simulink model "model"  (R2024b)
settings: Solver=ode1  StartTime=0.0  StopTime=10  FixedStep=0.0001  RelTol=1e-3
values from neighbouring files (symbols this model uses):
  a1 = c*a2    (= 810)    [init.m]
  a2 = c*a3    (= 270)    [init.m]
  a3 = c*a4    (= 90)    [init.m]
  a4 = c*10    (= 30)    [init.m]
  c1 = 50    [init.m]
  c2 = 1    [init.m]
  d = 100    [init.m]
  dis_gain = 30    [init.m]
  epsilon = 1    [init.m]
  i = 20    [init.m]
  k = 5    [init.m]
  mu = 0.9    [init.m]
  p = 400    [init.m]
  phi_frist = 0    [init.m]
  psi_frist = 0    [init.m]
  tau_p_max = 3000000    [init.m]
  theta_frist = 0    [init.m]
  umax = pi/2 - 0.01    (= 1.56079632679)    [init.m]
  w = wo    (= 50)    [init.m]
  wo = 50    [init.m]
  x_frist = 0    [init.m]
  y_frist = 0    [init.m]
  z_frist = 0    [init.m]
libraries: fod x36, slpidlib x6, simulink x1
(part 4 of 4)

== matlab function model/SMC/Subsystem/Subsystem6/MATLAB Function ==
  data: x input; z1_1 output; z1 input; z2 input; z3 input; z2_1 output; z3_1 output; z4 input; z4_1 output; a1 input; a2 input; a3 input; a4 input
function [z1_1,z2_1,z3_1,z4_1] = fcn(x,z1,z2,z3,z4,a1,a2,a3,a4)
    v1 = -a1*abs(z1-x)^(3/4)*sign(z1-x)+z2;
    z1_1 = v1;
    v2 = -a2*abs(z2-v1)^(2/3)*sign(z2-v1)+z3;
    z2_1 = v2;
    v3 = -a3*abs(z3-v2)^(1/2)*sign(z3-v2)+z4;
    z3_1 = v3;
    z4_1 = -a4*sign(z4-v3);
end

== matlab function model/MATLAB Function ==
  data: u input; y output
function y = fcn(u)

if u < 5
    y = 0;
else
    y = 1;
end

== matlab function model/系统5/MATLAB Function ==
  data: dnu output size=6*1; nu input; eta input; tau_p input; tau_d input; del input
function dnu = fcn(nu,eta,tau_p,tau_d,del)
    m = 5.5;
    I_x = 0.12;
    I_y = 0.25;
    I_z = 0.2;
    V = m;
    g = 9.8;

    x_B = 0;
    y_B = 0;
    z_B = -0.01;

    X_du = -2.61;
    K_dp = -0.15;
    X_u = -2.47;
    K_P = -0.82;
    X_uu = -8.33;
    K_pp = -2.95;
    Y_dv = -5.56;
    M_dq = -0.26;
    Y_v = -3.54;
    M_q = -0.9;
    Y_vv = -10.82;
    M_qq = -3.687;
    Z_dw = -9.75;
    N_dr = -0.21;
    Z_w = -2.38;
    N_r = -0.45;
    Z_ww = -14.13;
    N_rr = -1.56;

    m_u = m - X_du;
    m_v = m - Y_dv;
    m_w = m - Z_dw;
    m_p = I_x - K_dp;
    m_q = I_y - M_dq;
    m_r = I_z - N_dr;

    u = nu(1);
    v = nu(2);
    w = nu(3);
    p = nu(4);
    q = nu(5);
    r = nu(6);

    x = eta(1);
    y = eta(2);
    z = eta(3);
    phi = eta(4);
    theta = eta(5);
    psi = eta(6);

    M = [m_u 0 0 0 0 0;
         0 m_v 0 0 0 0;
         0 0 m_w 0 0 0;
         0 0 0 m_p 0 0;
         0 0 0 0 m_q 0;
         0 0 0 0 0 m_r];

    M = M+del*M;

    C = [0 0 0 0 m_w*w -m_r*v;
         0 0 0 -m_w*w 0 m_u*u;
         0 0 0 m_v*v -m_u*u 0;
         0 m_w*w -m_v*v 0 m_r*r -m_q*q;
         -m_w*w 0 m_u*u -m_r*r 0 m_p*p;
         m_v*v -m_u*u 0 m_q*q -m_p*p 0];

    C = C+del*C;
    
    D = -[X_uu*abs(u) 0 0 0 0 0;
          0 Y_vv*abs(v) 0 0 0 0;
          0 0 Z_ww*abs(w) 0 0 0;
          0 0 0 K_pp*abs(p) 0 0;
          0 0 0 0 M_qq*abs(q) 0;
          0 0 0 0 0 N_rr*abs(r)];

    D = D+del*D;
    
    B = g*V;

    g_eta = [0;0;0;-z_B*B*cos(theta)*sin(phi);-z_B*B*sin(theta);0];

    g_eta = g_eta+del*g_eta;

dnu = M\(tau_p + tau_d - C*nu - D*nu - g_eta);

== matlab function model/系统5/MATLAB Function1 ==
  data: eta input; deta output size=6*1; nv input
function deta = fcn(eta,nv)
    phi = eta(4);
    theta = eta(5);
    psi = eta(6);

    J =  [cos(psi)*cos(theta) -sin(psi)*cos(phi)+sin(phi)*sin(theta)*cos(psi) sin(psi)*sin(phi)+sin(theta)*cos(psi)*cos(phi) 0 0 0;
         sin(psi)*cos(theta) cos(psi)*cos(phi)+sin(phi)*sin(theta)*sin(psi) -cos(psi)*sin(phi)+sin(theta)*sin(psi)*cos(phi) 0 0 0;
         -sin(theta) sin(phi)*cos(theta) cos(psi)*cos(theta) 0 0 0;
         0 0 0 1 sin(phi)*tan(theta) cos(phi)*tan(theta);
         0 0 0 0 cos(phi) -sin(phi);
         0 0 0 0 sin(phi)/cos(theta) cos(phi)/cos(theta)];

deta = J*nv;

== matlab function model/ADRC/控制器/Subsystem1/Subsystem6/MATLAB Function2 ==
  data: h input; dh output size=3; eta input; tau_0 input; wo input
function dh = fcn(h,eta,tau_0,wo)

e = eta-h(1);

b1 = 3*wo;
b2  = 3*wo^2;
b3 = wo^3;

dh = [h(2)+b1*e;
    h(3)+b2*e+tau_0;
    b3*e;
    ];

== matlab function model/ADRC/控制器/Subsystem1/Subsystem1/MATLAB Function2 ==
  data: h input; dh output size=3; eta input; tau_0 input; wo input
function dh = fcn(h,eta,tau_0,wo)

e = eta-h(1);

b1 = 3*wo;
b2  = 3*wo^2;
b3 = wo^3;

dh = [h(2)+b1*e;
    h(3)+b2*e+tau_0;
    b3*e;
    ];

== matlab function model/FO_SMC_ESO/Levant微分器/Subsystem6/MATLAB Function ==
  data: x input; z1_1 output; z1 input; z2 input; z3 input; z2_1 output; z3_1 output; z4 input; z4_1 output; a1 input; a2 input; a3 input; a4 input
function [z1_1,z2_1,z3_1,z4_1] = fcn(x,z1,z2,z3,z4,a1,a2,a3,a4)
    v1 = -a1*abs(z1-x)^(3/4)*sign(z1-x)+z2;
    z1_1 = v1;
    v2 = -a2*abs(z2-v1)^(2/3)*sign(z2-v1)+z3;
    z2_1 = v2;
    v3 = -a3*abs(z3-v2)^(1/2)*sign(z3-v2)+z4;
    z3_1 = v3;
    z4_1 = -a4*sign(z4-v3);
end

== matlab function model/ADRC/控制器/Subsystem1/Subsystem2/MATLAB Function2 ==
  data: h input; dh output size=3; eta input; tau_0 input; wo input
function dh = fcn(h,eta,tau_0,wo)

e = eta-h(1);

b1 = 3*wo;
b2  = 3*wo^2;
b3 = wo^3;

dh = [h(2)+b1*e;
    h(3)+b2*e+tau_0;
    b3*e;
    ];

== matlab function model/ADRC/控制器/Subsystem1/Subsystem3/MATLAB Function2 ==
  data: h input; dh output size=3; eta input; tau_0 input; wo input
function dh = fcn(h,eta,tau_0,wo)

e = eta-h(1);

b1 = 3*wo;
b2  = 3*wo^2;
b3 = wo^3;

dh = [h(2)+b1*e;
    h(3)+b2*e+tau_0;
    b3*e;
    ];

== matlab function model/ADRC/控制器/Subsystem1/Subsystem4/MATLAB Function2 ==
  data: h input; dh output size=3; eta input; tau_0 input; wo input
function dh = fcn(h,eta,tau_0,wo)

e = eta-h(1);

b1 = 3*wo;
b2  = 3*wo^2;
b3 = wo^3;

dh = [h(2)+b1*e;
    h(3)+b2*e+tau_0;
    b3*e;
    ];

== matlab function model/ADRC/控制器/Subsystem1/Subsystem5/MATLAB Function2 ==
  data: h input; dh output size=3; eta input; tau_0 input; wo input
function dh = fcn(h,eta,tau_0,wo)

e = eta-h(1);

b1 = 3*wo;
b2  = 3*wo^2;
b3 = wo^3;

dh = [h(2)+b1*e;
    h(3)+b2*e+tau_0;
    b3*e;
    ];

== matlab function model/FO_SMC_ESO/MATLAB Function ==
  data: u1 input; y output; u2 input
function y = fcn(u1,u2)

y = u1+u2;

== matlab function model/eta_d_sin/MATLAB Function ==
  data: t input; y output
function y = fcn(t)
    
y = [3*sin(5*t);4*sin(5*t);5*sin(5*t)];
